simulink model "Lab4Ex2a(2)"  (R2023b)
settings: Solver=ode23tb  StartTime=0  StopTime=0.04  MaxStep=1/fpwm/200  RelTol=1e-3  AbsTol=1e-3
undefined symbols (not defined in the file): Cf, fpwm, Imin2, IoAVmin, kdv, kdv2, Ki, Kiv, Kp, Kpv, Lf, Po, Po2, Pomin, Pomin2, Rdv, Rdv2, ri, ri2, rLine, rLine2, Rmax, U, U2, ucmax, Vo, Vomax, Vomax2, Vomin, Vomin2
libraries: spsSeriesRLCBranchLib x12, spsVoltageMeasurementLib x7, spsCurrentMeasurementLib x6, spsMeanLib x6, spsBreakerLib x2, spsDiodeLib x2, spsMosfetLib x2, simulink x2, spsDCVoltageSourceLib x2, sps_lib x1
settings Model: Creator=ist1100080  LastModifiedBy=rodri
settings SolverCC: AutoScaleAbsTol=off  AlgebraicLoopSolver=TrustRegion  MaxZcPerStep=1
settings DebuggingCC: UnconnectedInputMsg=warning  UnconnectedOutputMsg=warning  UnconnectedLineMsg=warning  SymbolicDimsDataTypeCodeGenerationDiagnostic=none
settings ModelReferenceCC: EnableRefExpFcnMdlSchedulingChecks=on
settings SFSimCC: CustomCodeUndefinedFunction=UseInterfaceOnly
settings RTWCC: DLArmComputeVersion=19.05
settings SimscapeCC: SimscapeLogType=all  SimscapeLogSimulationStatistics=on  SimscapeLogDataHistory=10000

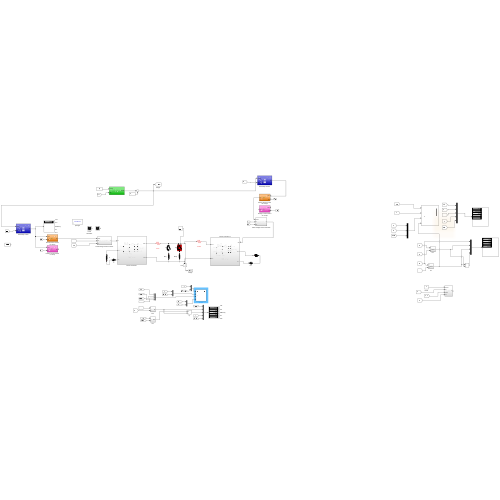
[thumbnail: Simulink's stored preview of the top-level diagram]
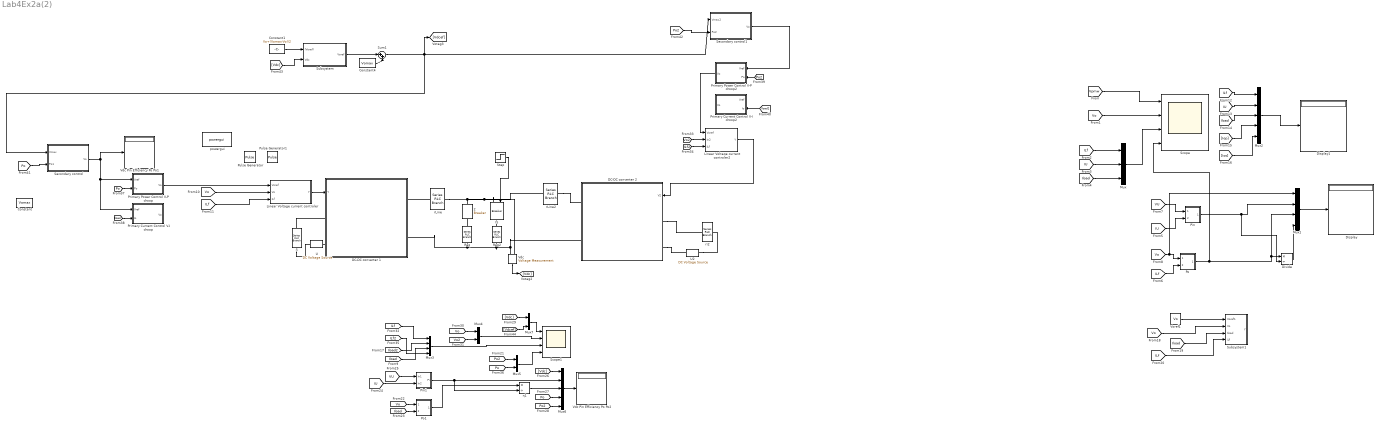
== system Lab4Ex2a(2) ==
  2 : spsBreakerLib/Breaker  InitialState=0  SwitchingTimes=[0.01]  External=off  BreakerResistance=0.01  SnubberResistance=Rs  SnubberCapacitance=Cs  Measurements=None  MoreParameters=on  NoBreakLoop=off
  Constant : Constant  Value=Vomax
  Constant1 : Constant  Value=Vo+(Vomax-Vo)/2
  Constant4 : Constant  Value=Vomax
  DC-DC converter 1 : Subsystem
  DC-DC converter 2 : Subsystem
  Display : Display
  Display1 : Display
  Divide : Product  Inputs=*/
  IS : spsBreakerLib/Breaker  InitialState=0  SwitchingTimes=[0.05]  External=on  BreakerResistance=0.01  SnubberResistance=Rs  SnubberCapacitance=Cs  Measurements=None  MoreParameters=on  NoBreakLoop=off
  Linear Voltage current controler : Subsystem
  Linear Voltage current controler2 : Subsystem
  Mux : Mux  Inputs=3
  Mux1 : Mux
  Mux2 : Mux  Inputs=5
  Mux3 : Mux
  Mux4 : Mux  Inputs=2
  Mux5 : Mux  Inputs=2
  Mux6 : Mux  Inputs=5
  Mux7 : Mux  Inputs=2
  Pin : Subsystem
  Pin1 : Subsystem
  Po : Subsystem
  Po1 : Subsystem
  Primary Current Control V-I droop : Subsystem
  Primary Current Control V-I droop2 : Subsystem
  Primary Power Control V-P droop : Subsystem
  Primary Power Control V-P droop2 : Subsystem
  Pulse Generator : DiscretePulseGenerator  PulseType=Time based  Period=1/fpwm  PulseWidth=48
  Pulse Generator1 : DiscretePulseGenerator  PulseType=Time based  Period=1/fpwm  PulseWidth=48
  Req : spsSeriesRLCBranchLib/Series RLC Branch  LConnTagsString=__new0  RConnTagsString=__new0  BranchType=R  Resistance=Rmax/14  Inductance=1e-3  SetiL0=off  InitialCurrent=0  Capacitance=1e-6  Setx0=off  InitialVoltage=0  Measurements=None
  Req2 : spsSeriesRLCBranchLib/Series RLC Branch  LConnTagsString=__new0  RConnTagsString=__new0  BranchType=R  Resistance=Rmax/18  Inductance=1e-3  SetiL0=off  InitialCurrent=0  Capacitance=1e-6  Setx0=off  InitialVoltage=0  Measurements=None
  Scope : Scope  NumInputPorts=4
  Scope1 : Scope  NumInputPorts=4
  Secondary control : Subsystem
  Secondary control1 : Subsystem
  Step : Step  Time=0.02  SampleTime=0
  Subsystem : Subsystem
  Subsystem1 : Subsystem
  Sum1 : Sum  Inputs=|++
  U : spsDCVoltageSourceLib/DC Voltage Source  Amplitude=U  Measurements=None
  U2 : spsDCVoltageSourceLib/DC Voltage Source  Amplitude=U2  Measurements=None
  Vdc : spsVoltageMeasurementLib/Voltage Measurement  PhasorSimulation=off  OutputType=Complex  PSBequivalent=0
  Vdc Pin Efficiency Po Po1 : Display
  Vdc Pin Efficiency Po Po2 : Display
  Voref1 : Constant  Value=Vo
  powergui : sps_lib/powergui  Priority=1  SimulationMode=Continuous  SampleTime=50e-6  frequency=60  Iterations=50  frequencyindice=0  Pbase=100e6  ErrMax=1e-4  UnitsV=kV  UnitsW=MW  buscounter=0  FunctionMessages=off  echomessages=off  EnableUseOfTLC=off  CurrentSourceSwitches=off  DisableSnubberDevices=off  DisableRonSwitches=off  DisableVfSwitches=off  DisplayEquations=off  AutomaticDiscreteSolvers=off  SolverType=Tustin/Backward Euler (TBE)  Interpol=off  ExternalGateDelay=off  methode=off  Ts=100  x0status=blocks  SPID=on  SwTol=0  HookPort=off  NonlinearTolerance=1e-4  nMaxIteration=100  ContinueOnMaxIteration=off  RestoreLinks=warning  ResistiveCurrentMeasurement=off  Frange=[0:2:500]  Ylog=off  Xlog=on  ShowGrid=off  save=off  variable=ZData  structure=0  ZoomFFT=off  StartTime=0.0  cycles=1  DisplayStyle=1  fundamental=60  FreqAxis=off  MaxFrequency=1000  frequencyindicesteady=1  RmsSteady=1  display=off
  rLine : spsSeriesRLCBranchLib/Series RLC Branch  LConnTagsString=__new0  RConnTagsString=__new0  BranchType=R  Resistance=rLine  Inductance=1e-3  SetiL0=off  InitialCurrent=0  Capacitance=1e-6  Setx0=off  InitialVoltage=0  Measurements=None
  rLine2 : spsSeriesRLCBranchLib/Series RLC Branch  LConnTagsString=__new0  RConnTagsString=__new0  BranchType=R  Resistance=rLine2  Inductance=1e-3  SetiL0=off  InitialCurrent=0  Capacitance=1e-6  Setx0=off  InitialVoltage=0  Measurements=None
  ri : spsSeriesRLCBranchLib/Series RLC Branch  LConnTagsString=__new0  RConnTagsString=__new0  BranchType=R  Resistance=ri  Inductance=1e-3  SetiL0=off  InitialCurrent=0  Capacitance=1e-6  Setx0=off  InitialVoltage=0  Measurements=None
  ri2 : spsSeriesRLCBranchLib/Series RLC Branch  LConnTagsString=__new0  RConnTagsString=__new0  BranchType=R  Resistance=ri2  Inductance=1e-3  SetiL0=off  InitialCurrent=0  Capacitance=1e-6  Setx0=off  InitialVoltage=0  Measurements=None
  ƞ1 : Product  Inputs=*/
  wires:
  [ILf] -> Mux/1
  [IU] -> Mux/2
  [Iload] -> Mux/3
  [VU] -> Pin/1(In1)
  [IU] -> Pin/2(In2)
  Pin/1(Mean1) -> Divide/2, Mux1/2
  [Vo] -> Mux1/1, Po/1(In1)
  [ILf] -> Po/2(In2)
  Po/1(Mean1) -> Scope/4, Mux1/3, Divide/1
  Divide/1 -> Mux1/4
  Mux1/1 -> Display/1
  Mux/1 -> Scope/3
  [Vpmw] -> Scope/1
  [Vo] -> Scope/2
  [Vo] -> Linear Voltage current controler/2(Vo)
  [ILf] -> Linear Voltage current controler/3(iLf)
  [Ios] -> Mux2/5
  [Iop] -> Mux2/4
  [IU] -> Mux2/2
  [Iload] -> Mux2/3
  [ILf] -> Mux2/1
  Mux2/1 -> Display1/1
  Voref1/1 -> Subsystem1/1(Voref1)
  [Vo] -> Subsystem1/2(Vo)
  [Iload] -> Subsystem1/3(Iload)
  [ILf] -> Subsystem1/4(iLf)
  Vdc/1 -> [Vdc]
  [Vo2] -> Linear Voltage current controler2/2(In2)
  [ILf2] -> Linear Voltage current controler2/3(iLf)
  Linear Voltage current controler2/1(Y) -> DC-DC converter 2/1(V2)
  [Iload] -> Po1/2(In2)
  [Po] -> Mux6/4
  [Vdc] -> Mux6/1
  [Po2] -> Mux6/5
  ƞ1/1 -> Mux6/3
  Mux3/1 -> Scope1/3
  Mux6/1 -> Vdc Pin Efficiency Po Po2/1
  [Vo] -> Po1/1(In1)
  [Iload] -> Mux3/3
  [Po2] -> Mux5/1
  Mux5/1 -> Scope1/4
  [ILf] -> Mux3/1
  [Vo] -> Mux4/1
  [Iload2] -> Mux3/2
  [Vo2] -> Mux4/2
  Mux4/1 -> Scope1/2
  [IU] -> Pin1/2(In2)
  [VU] -> Pin1/1(In1)
  Pin1/1(Pi) -> ƞ1/2, Mux6/2
  Po1/1(Po1) -> ƞ1/1
  Linear Voltage current controler/1(Y) -> DC-DC converter 1/1(Y)
  Step/1 -> IS/1
  [ILf2] -> Mux3/4
  [Po] -> Mux5/2
  [Po] -> Primary Power Control V-P droop/2(Po)
  [Iload] -> Primary Current Control V-I droop/2(Io)
  [Iload2] -> Primary Current Control V-I droop2/2(Io)
  [Po2] -> Primary Power Control V-P droop2/2(Po)
  Secondary control/1(Vo) -> Vdc Pin Efficiency Po Po1/1, Primary Current Control V-I droop/1(Vref), Primary Power Control V-P droop/1(Vref)
  [Po] -> Secondary control/2(Po1)
  [Po2] -> Secondary control1/2(Po2)
  Secondary control1/1(Vo) -> Primary Power Control V-P droop2/1(Vref)
  Primary Power Control V-P droop2/1(Vo) -> Linear Voltage current controler2/1(Voref)
  Primary Power Control V-P droop/1(Vo) -> Linear Voltage current controler/1(Voref)
  [Vdc] -> Subsystem/2(Vdc)
  Constant1/1 -> Subsystem/1((Voref))
  Subsystem/1(Voref) -> Sum1/1
  Constant4/1 -> Sum1/2
  Sum1/1 -> Secondary control1/1(Vmax2), Secondary control/1(Vmax), [Vdcef]
  [Vdc] -> Mux7/1
  Mux7/1 -> Scope1/1
  [Vdcef] -> Mux7/2
  connections:
  U/LConn1 -- DC-DC converter 1/LConn2
  rLine/RConn1 -- rLine2/LConn1 -- Vdc/LConn1 -- IS/LConn1 -- 2/LConn1
  Req2/RConn1 -- DC-DC converter 1/RConn2 -- Req/RConn1 -- DC-DC converter 2/RConn2 -- Vdc/LConn2
  Req2/LConn1 -- IS/RConn1
  Req/LConn1 -- 2/RConn1
  DC-DC converter 2/LConn2 -- U2/LConn1
  U2/RConn1 -- ri2/RConn1
  rLine2/RConn1 -- DC-DC converter 2/RConn1
  ri/LConn1 -- U/RConn1
  ri/RConn1 -- DC-DC converter 1/LConn1
  rLine/LConn1 -- DC-DC converter 1/RConn1
  DC-DC converter 2/LConn1 -- ri2/LConn1

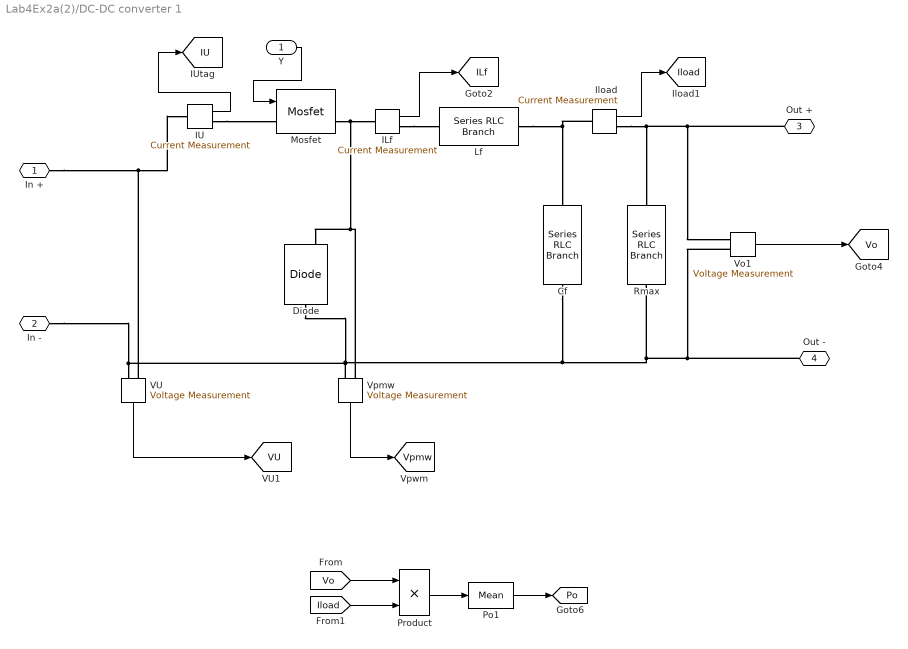
== system Lab4Ex2a(2)/DC-DC converter 1 ==
  Y : Inport
  Cf : spsSeriesRLCBranchLib/Series RLC Branch  LConnTagsString=__new0  RConnTagsString=__new0  BranchType=C  Resistance=1  Inductance=0  SetiL0=off  InitialCurrent=0  Capacitance=Cf  Setx0=on  InitialVoltage=Vo  Measurements=None
  Diode : spsDiodeLib/Diode  Ron=Ron  Lon=0  Vf=Vd  IC=0  UseSnubber=0  Rs=Rs  Cs=Cs  Measurements=on
  ILf : spsCurrentMeasurementLib/Current Measurement  PhasorSimulation=off  OutputType=Complex  PSBequivalent=0
  IU : spsCurrentMeasurementLib/Current Measurement  PhasorSimulation=off  OutputType=Complex  PSBequivalent=0
  Iload : spsCurrentMeasurementLib/Current Measurement  PhasorSimulation=off  OutputType=Complex  PSBequivalent=0
  Lf : spsSeriesRLCBranchLib/Series RLC Branch  LConnTagsString=__new0  RConnTagsString=__new0  BranchType=L  Resistance=1  Inductance=Lf  SetiL0=off  InitialCurrent=0  Capacitance=0  Setx0=off  InitialVoltage=0  Measurements=None
  Mosfet : spsMosfetLib/Mosfet  Ron=Ron  Lon=0  Rd=Rdson  Vfd=Vd  IC=0  Rs=Rs  Cs=Cs  Measurements=on
  Po1 : spsMeanLib/Mean  Freq=fpwm/10  Vinit=100  Ts=0
  Product : Product
  Rmax : spsSeriesRLCBranchLib/Series RLC Branch  LConnTagsString=__new0  RConnTagsString=__new0  BranchType=R  Resistance=Rmax  Inductance=0  SetiL0=off  InitialCurrent=0  Capacitance=0  Setx0=off  InitialVoltage=0  Measurements=None
  VU : spsVoltageMeasurementLib/Voltage Measurement  PhasorSimulation=off  OutputType=Complex  PSBequivalent=0
  Vo1 : spsVoltageMeasurementLib/Voltage Measurement  PhasorSimulation=off  OutputType=Complex  PSBequivalent=0
  Vpmw : spsVoltageMeasurementLib/Voltage Measurement  PhasorSimulation=off  OutputType=Complex  PSBequivalent=0
  In + : PMIOPort  Side=Left
  In - : PMIOPort  Port=2  Side=Left
  Out + : PMIOPort  Port=3  Side=Right
  Out - : PMIOPort  Port=4  Side=Right
  tag scope: ILf=global, IU=global, Iload=global, Po=global, VU=global, Vo=global, Vpmw=global
  wires:
  IU/1 -> [IU]
  VU/1 -> [VU]
  Vpmw/1 -> [Vpmw]
  ILf/1 -> [ILf]
  Iload/1 -> [Iload]
  Y/1 -> Mosfet/1
  Vo1/1 -> [Vo]
  Po1/1 -> [Po]
  [Iload] -> Product/2
  Product/1 -> Po1/1
  [Vo] -> Product/1
  connections:
  IU/RConn1 -- Mosfet/LConn1
  Lf/RConn1 -- Iload/LConn1 -- Cf/LConn1
  Diode/LConn1 -- Cf/RConn1 -- Out -/RConn1 -- Vo1/LConn2 -- Rmax/RConn1 -- Vpmw/LConn2 -- In -/RConn1 -- VU/LConn2
  Mosfet/RConn1 -- Diode/RConn1 -- Vpmw/LConn1 -- ILf/LConn1
  Iload/RConn1 -- Out +/RConn1 -- Vo1/LConn1 -- Rmax/LConn1
  ILf/RConn1 -- Lf/LConn1
  In +/RConn1 -- VU/LConn1 -- IU/LConn1

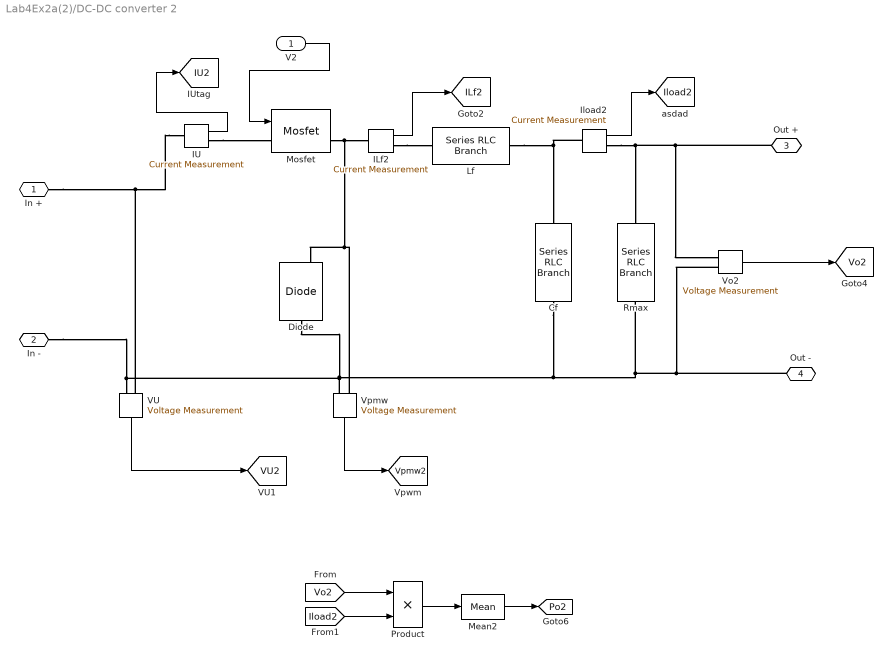
== system Lab4Ex2a(2)/DC-DC converter 2 ==
  V2 : Inport
  Cf : spsSeriesRLCBranchLib/Series RLC Branch  LConnTagsString=__new0  RConnTagsString=__new0  BranchType=C  Resistance=1  Inductance=0  SetiL0=off  InitialCurrent=0  Capacitance=Cf  Setx0=on  InitialVoltage=Vo  Measurements=None
  Diode : spsDiodeLib/Diode  Ron=Ron  Lon=0  Vf=Vd  IC=0  UseSnubber=0  Rs=Rs  Cs=Cs  Measurements=on
  ILf2 : spsCurrentMeasurementLib/Current Measurement  PhasorSimulation=off  OutputType=Complex  PSBequivalent=0
  IU : spsCurrentMeasurementLib/Current Measurement  PhasorSimulation=off  OutputType=Complex  PSBequivalent=0
  Iload2 : spsCurrentMeasurementLib/Current Measurement  PhasorSimulation=off  OutputType=Complex  PSBequivalent=0
  Lf : spsSeriesRLCBranchLib/Series RLC Branch  LConnTagsString=__new0  RConnTagsString=__new0  BranchType=L  Resistance=1  Inductance=Lf  SetiL0=off  InitialCurrent=0  Capacitance=0  Setx0=off  InitialVoltage=0  Measurements=None
  Mean2 : spsMeanLib/Mean  Freq=fpwm/10  Vinit=100  Ts=0
  Mosfet : spsMosfetLib/Mosfet  Ron=Ron  Lon=0  Rd=Rdson  Vfd=Vd  IC=0  Rs=Rs  Cs=Cs  Measurements=on
  Product : Product
  Rmax : spsSeriesRLCBranchLib/Series RLC Branch  LConnTagsString=__new0  RConnTagsString=__new0  BranchType=R  Resistance=Rmax  Inductance=0  SetiL0=off  InitialCurrent=0  Capacitance=0  Setx0=off  InitialVoltage=0  Measurements=None
  VU : spsVoltageMeasurementLib/Voltage Measurement  PhasorSimulation=off  OutputType=Complex  PSBequivalent=0
  Vo2 : spsVoltageMeasurementLib/Voltage Measurement  PhasorSimulation=off  OutputType=Complex  PSBequivalent=0
  Vpmw : spsVoltageMeasurementLib/Voltage Measurement  PhasorSimulation=off  OutputType=Complex  PSBequivalent=0
  In + : PMIOPort  Side=Left
  In - : PMIOPort  Port=2  Side=Left
  Out + : PMIOPort  Port=3  Side=Right
  Out - : PMIOPort  Port=4  Side=Right
  tag scope: ILf2=global, IU2=global, Iload2=global, Po2=global, VU2=global, Vo2=global, Vpmw2=global
  wires:
  IU/1 -> [IU2]
  VU/1 -> [VU2]
  Vpmw/1 -> [Vpmw2]
  ILf2/1 -> [ILf2]
  Iload2/1 -> [Iload2]
  Vo2/1 -> [Vo2]
  Mean2/1 -> [Po2]
  [Iload2] -> Product/2
  Product/1 -> Mean2/1
  [Vo2] -> Product/1
  V2/1 -> Mosfet/1
  connections:
  IU/RConn1 -- Mosfet/LConn1
  Lf/RConn1 -- Iload2/LConn1 -- Cf/LConn1
  VU/LConn2 -- Diode/LConn1 -- Cf/RConn1 -- Out -/RConn1 -- Vo2/LConn2 -- Rmax/RConn1 -- Vpmw/LConn2 -- In -/RConn1
  Mosfet/RConn1 -- Diode/RConn1 -- Vpmw/LConn1 -- ILf2/LConn1
  Iload2/RConn1 -- Out +/RConn1 -- Vo2/LConn1 -- Rmax/LConn1
  ILf2/RConn1 -- Lf/LConn1
  IU/LConn1 -- In +/RConn1 -- VU/LConn1

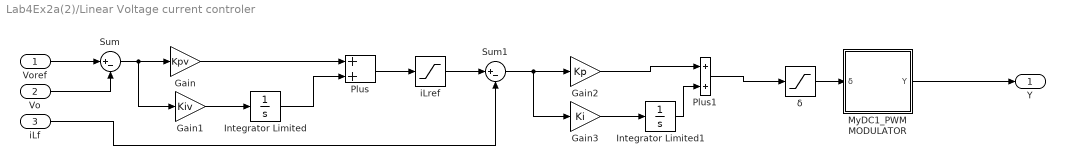
== system Lab4Ex2a(2)/Linear Voltage current controler ==
  Voref : Inport
  Vo : Inport  Port=2
  iLf : Inport  Port=3
  Gain : Gain  Gain=Kpv
  Gain1 : Gain  Gain=Kiv
  Gain2 : Gain  Gain=Kp
  Gain3 : Gain  Gain=Ki
  Integrator Limited : Integrator  LimitOutput=on  UpperSaturationLimit=1.3*Po/Vomin  LowerSaturationLimit=-1.3*Po/Vomin
  Integrator Limited1 : Integrator  LimitOutput=on  UpperSaturationLimit=1.3*Po/Vo  LowerSaturationLimit=-1.3*Po/Vo
  MyDC1_PWM MODULATOR : Subsystem
  Plus : Sum
  Plus1 : Sum
  Sum : Sum  Inputs=|+-
  Sum1 : Sum  Inputs=|+-
  iLref : Saturate  UpperLimit=1.3*Po/Vo  LowerLimit=-1.3*Po/Vo
  δ : Saturate  UpperLimit=0.99  LowerLimit=0.01
  Y : Outport
  wires:
  Plus1/1 -> δ/1
  Gain3/1 -> Integrator Limited1/1
  Voref/1 -> Sum/1
  Sum1/1 -> Gain3/1, Gain2/1
  Gain1/1 -> Integrator Limited/1
  Sum/1 -> Gain1/1, Gain/1
  iLf/1 -> Sum1/2
  Vo/1 -> Sum/2
  Integrator Limited/1 -> Plus/2
  Gain/1 -> Plus/1
  Gain2/1 -> Plus1/1
  δ/1 -> MyDC1_PWM MODULATOR/1(δ)
  Integrator Limited1/1 -> Plus1/2
  iLref/1 -> Sum1/1
  Plus/1 -> iLref/1
  MyDC1_PWM MODULATOR/1(Y) -> Y/1

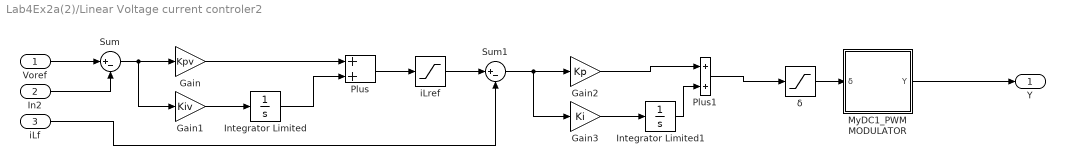
== system Lab4Ex2a(2)/Linear Voltage current controler2 ==
  Voref : Inport
  In2 : Inport  Port=2
  iLf : Inport  Port=3
  Gain : Gain  Gain=Kpv
  Gain1 : Gain  Gain=Kiv
  Gain2 : Gain  Gain=Kp
  Gain3 : Gain  Gain=Ki
  Integrator Limited : Integrator  LimitOutput=on  UpperSaturationLimit=1.3*Po/Vo  LowerSaturationLimit=-1.3*Po/Vo
  Integrator Limited1 : Integrator  LimitOutput=on  UpperSaturationLimit=1.3*Po/Vo  LowerSaturationLimit=-1.3*Po/Vo
  MyDC1_PWM MODULATOR : Subsystem
  Plus : Sum
  Plus1 : Sum
  Sum : Sum  Inputs=|+-
  Sum1 : Sum  Inputs=|+-
  iLref : Saturate  UpperLimit=1.3*Po/Vo  LowerLimit=-1.3*Po/Vo
  δ : Saturate  UpperLimit=0.99  LowerLimit=0.01
  Y : Outport
  wires:
  Plus1/1 -> δ/1
  Gain3/1 -> Integrator Limited1/1
  Voref/1 -> Sum/1
  Sum1/1 -> Gain3/1, Gain2/1
  Gain1/1 -> Integrator Limited/1
  Sum/1 -> Gain1/1, Gain/1
  iLf/1 -> Sum1/2
  In2/1 -> Sum/2
  Integrator Limited/1 -> Plus/2
  Gain/1 -> Plus/1
  Gain2/1 -> Plus1/1
  δ/1 -> MyDC1_PWM MODULATOR/1(δ)
  Integrator Limited1/1 -> Plus1/2
  iLref/1 -> Sum1/1
  Plus/1 -> iLref/1
  MyDC1_PWM MODULATOR/1(Y) -> Y/1

== system Lab4Ex2a(2)/Pin ==
  In1 : Inport
  In2 : Inport  Port=2
  Mean : spsMeanLib/Mean  Freq=0.1*fpwm  Vinit=110  Ts=0
  Product : Product
  Mean1 : Outport
  wires:
  Product/1 -> Mean/1
  In2/1 -> Product/2
  In1/1 -> Product/1
  Mean/1 -> Mean1/1

== system Lab4Ex2a(2)/Pin1 ==
  In1 : Inport
  In2 : Inport  Port=2
  Mean : spsMeanLib/Mean  Freq=0.1*fpwm  Vinit=110  Ts=0
  Product : Product
  Pi : Outport
  wires:
  Product/1 -> Mean/1
  In2/1 -> Product/2
  In1/1 -> Product/1
  Mean/1 -> Pi/1

== system Lab4Ex2a(2)/Po ==
  In1 : Inport
  In2 : Inport  Port=2
  Mean : spsMeanLib/Mean  Freq=0.1*fpwm  Vinit=110  Ts=0
  Product : Product
  Mean1 : Outport
  wires:
  Product/1 -> Mean/1
  In2/1 -> Product/2
  In1/1 -> Product/1
  Mean/1 -> Mean1/1

== system Lab4Ex2a(2)/Po1 ==
  In1 : Inport
  In2 : Inport  Port=2
  Mean : spsMeanLib/Mean  Freq=0.1*fpwm  Vinit=110  Ts=0
  Product : Product
  Po1 : Outport
  wires:
  Product/1 -> Mean/1
  In2/1 -> Product/2
  In1/1 -> Product/1
  Mean/1 -> Po1/1

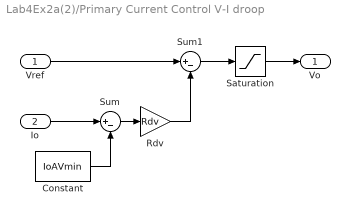
== system Lab4Ex2a(2)/Primary Current Control V-I droop ==
  Vref : Inport
  Io : Inport  Port=2
  Constant : Constant  Value=IoAVmin
  Rdv : Gain  Gain=Rdv
  Saturation : Saturate  UpperLimit=Vomax+1  LowerLimit=Vomin-1
  Sum : Sum  Inputs=|+-
  Sum1 : Sum  Inputs=|+-
  Vo : Outport
  wires:
  Constant/1 -> Sum/2
  Vref/1 -> Sum1/1
  Io/1 -> Sum/1
  Rdv/1 -> Sum1/2
  Sum1/1 -> Saturation/1
  Saturation/1 -> Vo/1
  Sum/1 -> Rdv/1

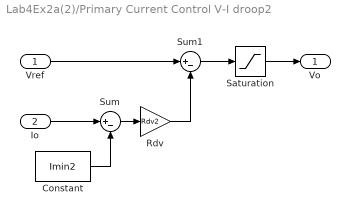
== system Lab4Ex2a(2)/Primary Current Control V-I droop2 ==
  Vref : Inport
  Io : Inport  Port=2
  Constant : Constant  Value=Imin2
  Rdv : Gain  Gain=Rdv2
  Saturation : Saturate  UpperLimit=Vomax2+1  LowerLimit=Vomin2-1
  Sum : Sum  Inputs=|+-
  Sum1 : Sum  Inputs=|+-
  Vo : Outport
  wires:
  Constant/1 -> Sum/2
  Vref/1 -> Sum1/1
  Io/1 -> Sum/1
  Rdv/1 -> Sum1/2
  Sum1/1 -> Saturation/1
  Saturation/1 -> Vo/1
  Sum/1 -> Rdv/1

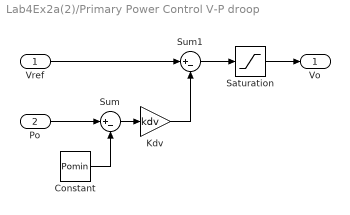
== system Lab4Ex2a(2)/Primary Power Control V-P droop ==
  Vref : Inport
  Po : Inport  Port=2
  Constant : Constant  Value=Pomin
  Kdv : Gain  Gain=kdv
  Saturation : Saturate  UpperLimit=Vomax+1  LowerLimit=Vomin-1
  Sum : Sum  Inputs=|+-
  Sum1 : Sum  Inputs=|+-
  Vo : Outport
  wires:
  Constant/1 -> Sum/2
  Po/1 -> Sum/1
  Sum/1 -> Kdv/1
  Kdv/1 -> Sum1/2
  Vref/1 -> Sum1/1
  Sum1/1 -> Saturation/1
  Saturation/1 -> Vo/1

== system Lab4Ex2a(2)/Primary Power Control V-P droop2 ==
  Vref : Inport
  Po : Inport  Port=2
  Constant : Constant  Value=Pomin2
  Kdv : Gain  Gain=kdv2
  Saturation : Saturate  UpperLimit=Vomax2+1  LowerLimit=Vomin-1
  Sum : Sum  Inputs=|+-
  Sum1 : Sum  Inputs=|+-
  Vo : Outport
  wires:
  Constant/1 -> Sum/2
  Po/1 -> Sum/1
  Sum/1 -> Kdv/1
  Kdv/1 -> Sum1/2
  Vref/1 -> Sum1/1
  Sum1/1 -> Saturation/1
  Saturation/1 -> Vo/1

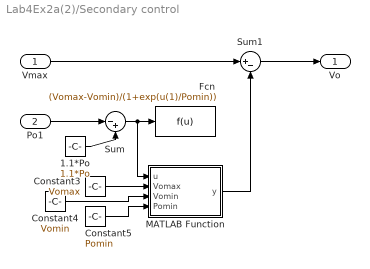
== system Lab4Ex2a(2)/Secondary control ==
  Vmax : Inport
  Po1 : Inport  Port=2
  1.1*Po : Constant  Value=1.1*Po
  Constant3 : Constant  Value=Vomax
  Constant4 : Constant  Value=Vomin
  Constant5 : Constant  Value=Pomin
  Fcn : Fcn  Expr=(Vomax-Vomin)/(1+exp(u(1)/Pomin))
  MATLAB Function : MATLAB Function  TreatAsAtomicUnit=on
  Sum : Sum  Inputs=|-+
  Sum1 : Sum  Inputs=|+-
  Vo : Outport
  wires:
  Constant5/1 -> MATLAB Function/4(Pomin)
  Sum1/1 -> Vo/1
  Sum/1 -> MATLAB Function/1(u), Fcn/1
  Po1/1 -> Sum/1
  Vmax/1 -> Sum1/1
  MATLAB Function/1(y) -> Sum1/2
  1.1*Po/1 -> Sum/2
  Constant3/1 -> MATLAB Function/2(Vomax)
  Constant4/1 -> MATLAB Function/3(Vomin)

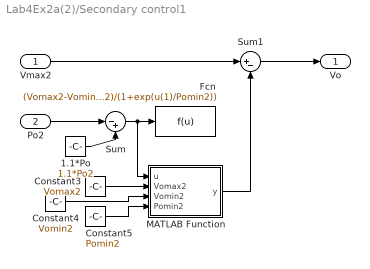
== system Lab4Ex2a(2)/Secondary control1 ==
  Vmax2 : Inport
  Po2 : Inport  Port=2
  1.1*Po : Constant  Value=1.1*Po2
  Constant3 : Constant  Value=Vomax2
  Constant4 : Constant  Value=Vomin2
  Constant5 : Constant  Value=Pomin2
  Fcn : Fcn  Expr=(Vomax2-Vomin2)/(1+exp(u(1)/Pomin2))
  MATLAB Function : MATLAB Function  TreatAsAtomicUnit=on
  Sum : Sum  Inputs=|-+
  Sum1 : Sum  Inputs=|+-
  Vo : Outport
  wires:
  Constant5/1 -> MATLAB Function/4(Pomin2)
  Sum1/1 -> Vo/1
  Sum/1 -> MATLAB Function/1(u), Fcn/1
  Po2/1 -> Sum/1
  Vmax2/1 -> Sum1/1
  MATLAB Function/1(y) -> Sum1/2
  1.1*Po/1 -> Sum/2
  Constant3/1 -> MATLAB Function/2(Vomax2)
  Constant4/1 -> MATLAB Function/3(Vomin2)

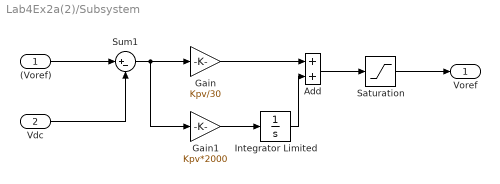
== system Lab4Ex2a(2)/Subsystem ==
  (Voref) : Inport
  Vdc : Inport  Port=2
  Add : Sum
  Gain : Gain  Gain=Kpv/30
  Gain1 : Gain  Gain=Kpv*2000
  Integrator Limited : Integrator  LimitOutput=on  UpperSaturationLimit=(Vomax-Vo)/2  LowerSaturationLimit=-(Vomax-Vo)/2
  Saturation : Saturate  UpperLimit=(Vomax-Vo)/2  LowerLimit=-(Vomax-Vo)/2
  Sum1 : Sum  Inputs=|+-
  Voref : Outport
  wires:
  Add/1 -> Saturation/1
  Integrator Limited/1 -> Add/2
  Vdc/1 -> Sum1/2
  Sum1/1 -> Gain1/1, Gain/1
  Saturation/1 -> Voref/1
  Gain/1 -> Add/1
  Gain1/1 -> Integrator Limited/1
  (Voref)/1 -> Sum1/1

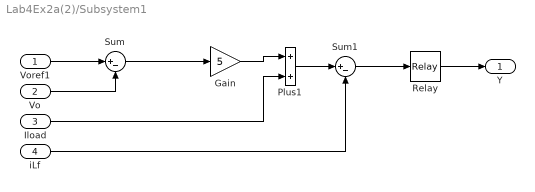
== system Lab4Ex2a(2)/Subsystem1 ==
  Voref1 : Inport
  Vo : Inport  Port=2
  Iload : Inport  Port=3
  iLf : Inport  Port=4
  Gain : Gain  Gain=5
  Plus1 : Sum
  Relay : Relay  OnSwitchValue=IoAVmin/2  OffSwitchValue=-IoAVmin/2
  Sum : Sum  Inputs=|+-
  Sum1 : Sum  Inputs=|+-
  Y : Outport
  wires:
  Vo/1 -> Sum/2
  Sum/1 -> Gain/1
  Relay/1 -> Y/1
  Plus1/1 -> Sum1/1
  iLf/1 -> Sum1/2
  Sum1/1 -> Relay/1
  Gain/1 -> Plus1/1
  Voref1/1 -> Sum/1
  Iload/1 -> Plus1/2

== system Lab4Ex2a(2)/Linear Voltage current controler/MyDC1_PWM MODULATOR ==
  δ : Inport
  Relay : Relay  OnSwitchValue=0.01  OffSwitchValue=-0.01
  Repeating Sequence : simulink/Sources/Repeating Sequence  rep_seq_t=[0 1/fpwm]  rep_seq_y=[0 ucmax]
  Sum2 : Sum  Inputs=|+-
  Y : Outport
  wires:
  Repeating Sequence/1 -> Sum2/2
  δ/1 -> Sum2/1
  Sum2/1 -> Relay/1
  Relay/1 -> Y/1

== system Lab4Ex2a(2)/Linear Voltage current controler2/MyDC1_PWM MODULATOR ==
  δ : Inport
  Relay : Relay  OnSwitchValue=0.01  OffSwitchValue=-0.01
  Repeating Sequence : simulink/Sources/Repeating Sequence  rep_seq_t=[0 1/fpwm]  rep_seq_y=[0 ucmax]
  Sum2 : Sum  Inputs=|+-
  Y : Outport
  wires:
  Repeating Sequence/1 -> Sum2/2
  δ/1 -> Sum2/1
  Sum2/1 -> Relay/1
  Relay/1 -> Y/1

== matlab function Lab4Ex2a(2)/Secondary control1/MATLAB Function ==
  data: u input; y output; Vomax2 input; Vomin2 input; Pomin2 input
function y = fcn(u, Vomax2, Vomin2, Pomin2)

y = (Vomax2-Vomin2)/(1+exp(u/Pomin2));

== matlab function Lab4Ex2a(2)/Secondary control/MATLAB Function ==
  data: u input; y output; Vomax input; Vomin input; Pomin input
function y = fcn(u, Vomax, Vomin, Pomin)

y = (Vomax-Vomin)/(1+exp(u/Pomin));
